simulink model "a_20210531_test_GPS"  (R2020b)
settings: Solver=FixedStepDiscrete  StartTime=0.0  StopTime=inf  FixedStep=0.01  RelTol=1e-3  EnableMultiTasking=on
libraries: arduinolib x2
settings Model: SimulationMode=external  SILPILModeSetting=veronly  ExtModeTrigDuration=2  Creator=alexv  LastModifiedBy=lapis-dspace
settings OptimizationCC: EnhancedBackFolding=on  PassReuseOutputArgsAs=Individual arguments  ZeroExternalMemoryAtStartup=off  ZeroInternalMemoryAtStartup=off  MaxStackSize=64  OptimizeBlockOrder=speed  DifferentSizesBufferReuse=on  OptimizationCustomize=off  EfficientTunableParamExpr=on
settings DebuggingCC: ParameterTunabilityLossMsg=error
settings HardwareCC: ProdBitPerPointer=32  ProdBitPerSizeT=32  ProdBitPerPtrDiffT=32  ProdLargestAtomicInteger=Long  ProdLargestAtomicFloat=Double  ProdWordSize=32  ProdHWDeviceType=ARM Compatible->ARM Cortex
settings SFSimCC: MATLABDynamicMemAlloc=off
settings RTWCC: Description=Embedded Coder  SystemTargetFile=ert.tlc  HardwareBoard=Arduino Due  TemplateMakefile=ert_default_tmf  Toolchain=Arduino ARM  BuildConfiguration=Faster Runs
settings CodeAppCC: ForceParamTrailComments=on  IgnoreCustomStorageClasses=off  OperatorAnnotations=on  SimulinkDataObjDesc=on  SFDataObjDesc=on  InsertBlockDesc=on
settings ERTTargetCC: SupportContinuousTime=on  SupportVariableSizeSignals=on  ExtModeTransport=3  ExtModeStaticAllocSize=24576  ExtModeMexFile=ext_xcp  ExtModeIntrfLevel=Level2 - Open

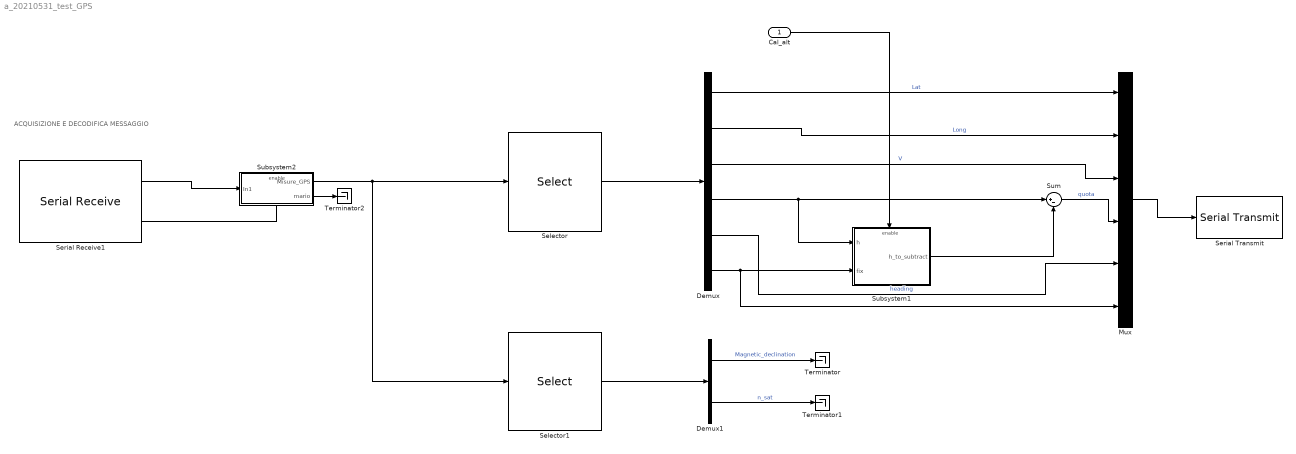
== system a_20210531_test_GPS ==
  note: ACQUISIZIONE E DECODIFICA MESSAGGIO
  Cal_alt : Inport
  Demux : Demux  Outputs=6
  Demux1 : Demux  Outputs=2
  Mux : Mux  Inputs=6
  Selector : Selector  InputPortWidth=9  IndexOptions=Index vector (dialog)  Indices=[1 2 3 8 5 6]  OutputSizes=1
  Selector1 : Selector  InputPortWidth=9  IndexOptions=Index vector (dialog)  Indices=[4 7]  OutputSizes=1
  Serial Receive1 : arduinolib/Serial Receive  isARMArch=on  portNumber=1  DataType=uint8  Datalength=32  SampleTime=0.01  showOutStatus=on  blockPlatform=arduino
      settings: SourceProductBaseCode=ARDUINO
  Serial Transmit : arduinolib/Serial Transmit  portNumber=0  sendmode=println  sendformat=Decimal  floatprecision=2  blockPlatform=arduino
  Subsystem1 : Subsystem
  Subsystem2 : Subsystem
  Sum : Sum  Inputs=|+-
  Terminator : Terminator
  Terminator1 : Terminator
  Terminator2 : Terminator
  wires:
  Demux1/2 -> Terminator1/1  "n_sat"
  Demux1/1 -> Terminator/1  "Magnetic_declination"
  Subsystem2/2(mario) -> Terminator2/1
  Selector/1 -> Demux/1
  Mux/1 -> Serial Transmit/1
  Demux/2 -> Mux/2  "Long"
  Sum/1 -> Mux/4  "quota"
  Serial Receive1/1 -> Subsystem2/1(In1)
  Cal_alt/1 -> Subsystem1/Enable
  Demux/3 -> Mux/3  "V"
  Demux/5 -> Mux/5  "heading"
  Subsystem1/1(h_to_subtract) -> Sum/2
  Selector1/1 -> Demux1/1
  Demux/1 -> Mux/1  "Lat"
  Demux/4 -> Sum/1, Subsystem1/1(h)
  Serial Receive1/2 -> Subsystem2/Enable
  Subsystem2/1(Misure_GPS) -> Selector/1, Selector1/1
  Demux/6 -> Mux/6, Subsystem1/2(fix)

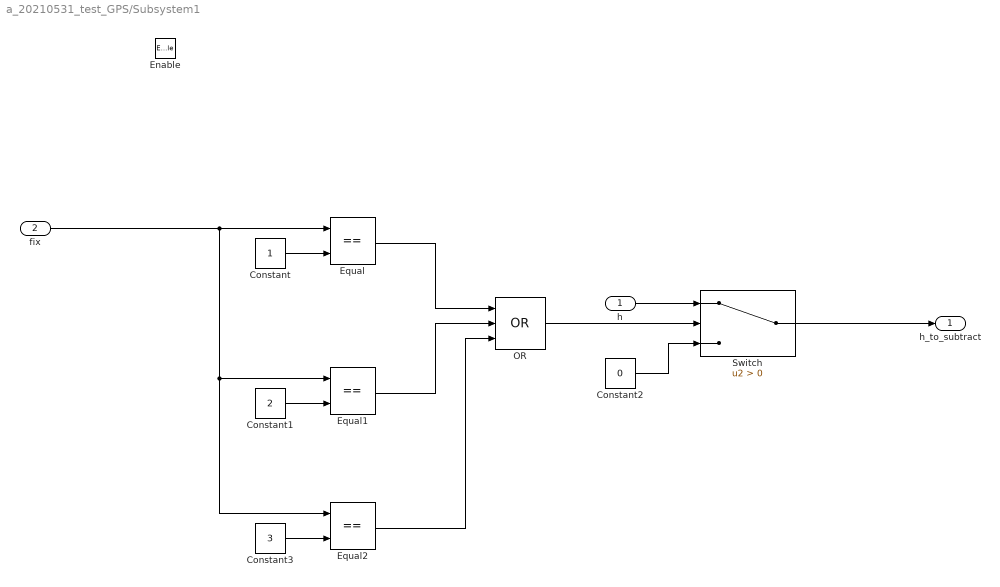
== system a_20210531_test_GPS/Subsystem1 ==
  h : Inport
  fix : Inport  Port=2
  Enable : EnablePort
  Constant : Constant
  Constant1 : Constant  Value=2
  Constant2 : Constant  Value=0
  Constant3 : Constant  Value=3
  Equal : RelationalOperator  Operator===  OutDataTypeStr=boolean  RndMeth=Simplest
  Equal1 : RelationalOperator  Operator===  OutDataTypeStr=boolean  RndMeth=Simplest
  Equal2 : RelationalOperator  Operator===  OutDataTypeStr=boolean  RndMeth=Simplest
  OR : Logic  Operator=OR  Inputs=3  IconShape=distinctive  AllPortsSameDT=off  OutDataTypeStr=boolean
  Switch : Switch  Criteria=u2 > Threshold
  h_to_subtract : Outport  VectorParamsAs1DForOutWhenUnconnected=off
  wires:
  Constant/1 -> Equal/2
  Equal/1 -> OR/1
  Constant1/1 -> Equal1/2
  Equal1/1 -> OR/2
  h/1 -> Switch/1
  OR/1 -> Switch/2
  Constant2/1 -> Switch/3
  Switch/1 -> h_to_subtract/1
  Equal2/1 -> OR/3
  Constant3/1 -> Equal2/2
  fix/1 -> Equal2/1, Equal1/1, Equal/1

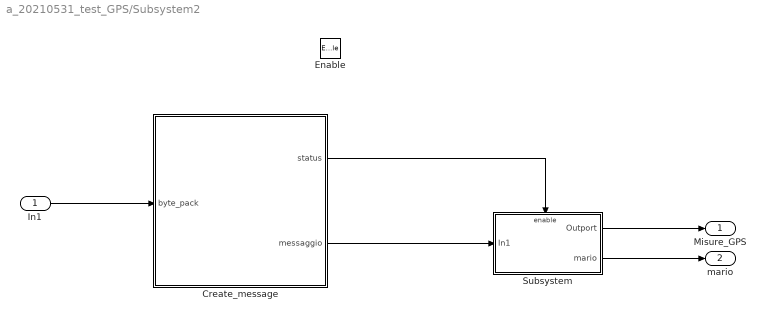
== system a_20210531_test_GPS/Subsystem2 ==
  In1 : Inport
  Enable : EnablePort
  Create_message : MATLAB Function  TreatAsAtomicUnit=on
  Subsystem : Subsystem
  Misure_GPS : Outport  VectorParamsAs1DForOutWhenUnconnected=off
  mario : Outport  Port=2  VectorParamsAs1DForOutWhenUnconnected=off
  wires:
  In1/1 -> Create_message/1(byte_pack)
  Create_message/1(status) -> Subsystem/Enable
  Subsystem/2(mario) -> mario/1
  Create_message/2(messaggio) -> Subsystem/1(In1)
  Subsystem/1(Outport) -> Misure_GPS/1

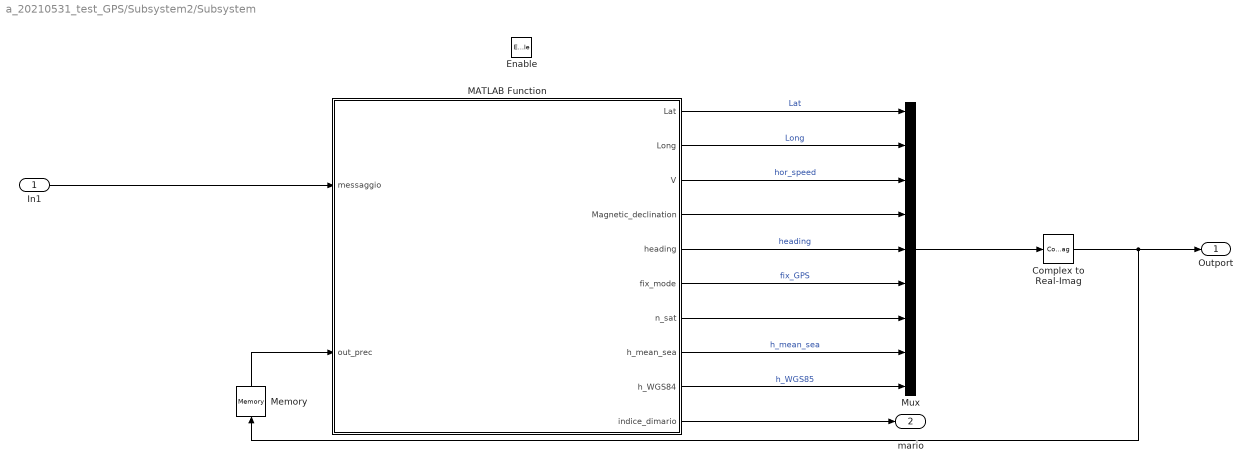
== system a_20210531_test_GPS/Subsystem2/Subsystem ==
  In1 : Inport
  Enable : EnablePort
  Complex to Real-Imag : ComplexToRealImag  Output=Real
  MATLAB Function : MATLAB Function  TreatAsAtomicUnit=on
  Memory : Memory  InheritSampleTime=on
  Mux : Mux  Inputs=9
  Outport : Outport  VectorParamsAs1DForOutWhenUnconnected=off
  mario : Outport  Port=2  VectorParamsAs1DForOutWhenUnconnected=off
  wires:
  MATLAB Function/2(Long) -> Mux/2  "Long"
  Memory/1 -> MATLAB Function/2(out_prec)
  MATLAB Function/8(h_mean_sea) -> Mux/8  "h_mean_sea"
  MATLAB Function/3(V) -> Mux/3  "hor_speed"
  MATLAB Function/1(Lat) -> Mux/1  "Lat"
  Mux/1 -> Complex to Real-Imag/1
  MATLAB Function/9(h_WGS84) -> Mux/9  "h_WGS85"
  MATLAB Function/5(heading) -> Mux/5  "heading"
  MATLAB Function/6(fix_mode) -> Mux/6  "fix_GPS"
  MATLAB Function/4(Magnetic_declination) -> Mux/4
  MATLAB Function/7(n_sat) -> Mux/7
  In1/1 -> MATLAB Function/1(messaggio)
  MATLAB Function/10(indice_dimario) -> mario/1
  Complex to Real-Imag/1 -> Memory/1, Outport/1

== matlab function a_20210531_test_GPS/Subsystem2/Create_message ==
  data: status output; byte_pack input; messaggio output
function [status,messaggio]  = LETTURA_NMEA(byte_pack)

persistent message counter start_found end_found

status = false;       %ho aggiunto questo
messaggio = uint8(zeros(1,80)) ;
pos_end = uint8(0) ;
M = uint8(length(byte_pack)) ;


if isempty(end_found) 
    end_found = false ;
end 
if isempty(start_found) 
     start_found = false ;
end 
if isempty (counter) 
    counter = uint8(0) ;
end 
if isempty(message)
     message = uint8(zeros(1,80)) ;
end



if start_found == 0 
    for i = uint8(1) : M  
        if byte_pack(i) == '$' 
            message(1:M - (i-1)) = byte_pack(i:end) ;
            counter = M - (i-1) ; 
            start_found = true ;
            break
        end
    end
    
    
elseif start_found == 1
    for i = uint8(1) : M  
        if byte_pack(i) == 13 
            end_found = true ;
            pos_end = i ;
            break
        end
    end
    
    if end_found == 1
        message(counter + 1 : counter + pos_end) = byte_pack(1:pos_end) ;
        status = true;       %ho aggiunto questo
        messaggio = message ;
        end_found = false ;
        counter = M - pos_end ;
        if pos_end == M 
            start_found = false ; 
            message = uint8(zeros(1,80)) ;
        else  
            start_found = true ;
            message(1:(M - pos_end)) = byte_pack(pos_end + 1 : end) ;
            message(M - pos_end +1 : 80) = uint8(zeros(1,80 - (M - pos_end) )) ;
        end
         

    else 
    message(counter + 1 : M + counter ) = byte_pack ;
    counter = M + counter  ;
   
    end
    
    
 
        
    
    
end

== matlab function a_20210531_test_GPS/Subsystem2/Subsystem/MATLAB Function ==
  data: messaggio input; Lat output; Long output; V output; Magnetic_declination output; heading output; fix_mode output; n_sat output; h_mean_sea output; h_WGS84 output; out_prec input; indice_dimario output
function [Lat,Long,V,Magnetic_declination,heading,fix_mode,n_sat,h_mean_sea,h_WGS84,indice_dimario] = parser_NMEA(messaggio,out_prec)


messaggio = char(messaggio) ;

comma_gga = uint8(zeros(1,14));
comma_rmc = uint8(zeros(1,12));
star = uint8(0);
dollar = uint8(0);
find_dollar = uint8(0);
find_comma = uint8(0);
message_type = uint8(zeros(1,5));
indice_dimario = uint8(0);





for i=1:length(messaggio)
    if messaggio(i) == '$'
        find_dollar = find_dollar + uint8(1);
    end
    if messaggio(i) == ','
        find_comma = find_comma + uint8(1);
    end
end

if (find_dollar == 1 && (find_comma == 12 || find_comma == 14))              % controllo se il numero di $ e , sono corretti all'interno di messaggio
    % altrimenti il messaggio è corrotto ed in output mando i messaggi
    % precedenti
    dollar= find(messaggio == '$',1);
    
    mess_type = messaggio(dollar(1) + 1 : dollar(1) + 5);                        % è il nome del messaggio arrivato
    
    % decodifica mesaggio RMC
    
    if mess_type == 'GPRMC'                                                          %esempio per i bimbi stupidi come noi: $GPRMC,081836,A,3751.65,S,14507.36,E,000.0,360.0,130998,011.3,E*62
        comma_rmc = find(messaggio == ',');                                          % restituisce le posizioni delle virgole all'interno del messaggio
        star = find(messaggio == '*');                                               % restituisce la posizione dell'asterisco all'interno del messaggio
        dollar = find(messaggio == '$');                                             % restituisce la posizione del dollaro all'interno del messaggio
        
        Lat_1 = str2double(messaggio(comma_rmc(3) + 1 : comma_rmc(3) + 2));
        Lat_2 = str2double(messaggio(comma_rmc(3) + 3 : comma_rmc(4) - 1))/60;
        Lat = Lat_1 + Lat_2;
        if messaggio(comma_rmc(4) + 1) == 'S'
            Lat = -Lat;
        end
        
        
        Long_1 = str2double(messaggio(comma_rmc(5) + 1 : comma_rmc(5) + 3));
        Long_2 = str2double(messaggio(comma_rmc(5) + 4 : comma_rmc(6) - 1))/60;
        Long = Long_1 + Long_2;
        if messaggio(comma_rmc(6) + 1) == 'W'
            Long = -Long;
        end
        
        V = str2double(messaggio(comma_rmc(7) + 1 : comma_rmc(8) - 1));
        
        heading = str2double(messaggio(comma_rmc(8) + 1 : comma_rmc(9) - 1));
        
        Magnetic_declination = str2double(messaggio(comma_rmc(10) + 1 : comma_rmc(11) - 1));
        if messaggio(comma_rmc(11) + 1) == 'W'
            Magnetic_declination = -Magnetic_declination;
        end
        
        % questi dati non sono presenti nel messaggio rmc, quindi prendo quelli
        % precedenti
        
        fix_mode = complex(out_prec(6),0);
        
        n_sat = complex(out_prec(7),0) ;
        
        h_mean_sea = complex(out_prec(8),0) ;
        
        h_WGS84 = complex(out_prec(9),0) ;
        
        
        %%%%%%%%%%%%%%%%%%%%%%%%%%%%%%%%%%%%%%%%%%%%%%%%%%%%%%%%%
        
        % calcolo checksum
        
        ck_ric = char(zeros(1,2)) ;
        ck_ric(1) = messaggio(star(1) + uint8(1))  ;
        ck_ric(2) = messaggio(star(1) + uint8(2)) ;
        
        NMEA_rmc_string = uint8(messaggio(dollar(1)+1:star(1)-1)) ;
        
        checksum = uint8(0) ;
        for i = 1:length(NMEA_rmc_string)
            checksum = bitxor(checksum,NMEA_rmc_string(i),'uint8') ;
        end
        
        if checksum ~= hex2dec(ck_ric)
            Lat = out_prec(1) ;
            Long = out_prec(2) ;
            V = out_prec(3) ;
            Magnetic_declination = out_prec(4);
            heading = out_prec(5) ;
            fix_mode = complex(out_prec(6),0);
            n_sat = complex(out_prec(7),0) ;
            h_mean_sea = complex(out_prec(8),0) ;
            h_WGS84 = complex(out_prec(9),0) ;
            indice_dimario = uint8(10);
        end
        
        %%%%%%%%%%%%%%%%%%%%%%%%%%%%%%%%%%%%%%%%%%%%%%%%%%%%%%%%%%%
        
        % decodifica mesaggio GGA
        
    elseif mess_type == 'GPGGA'
        comma_gga = find(messaggio == ',');
        star = find(messaggio == '*');
        dollar = find(messaggio == '$');
        
        
        Lat_1 = str2double(messaggio(comma_gga(2) + 1 : comma_gga(2) + 2));
        Lat_2 = str2double(messaggio(comma_gga(2) + 3 : comma_gga(3) - 1))/60;
        Lat = Lat_1 + Lat_2;
        if messaggio(comma_gga(3) + 1) == 'S'
            Lat = -Lat;
        end
        
        
        Long_1 = str2double(messaggio(comma_gga(4) + 1 : comma_gga(4) + 3));
        Long_2 = str2double(messaggio(comma_gga(4) + 4 : comma_gga(5) - 1))/60;
        Long = Long_1 + Long_2;
        if messaggio(comma_gga(5) + 1) == 'W'
            Long = -Long;
        end
        
        
        fix_mode = str2double(messaggio(comma_gga(6) + 1));
        
        n_sat = str2double(messaggio(comma_gga(7) + 1 : comma_gga(8) - 1));
        
        h_mean_sea = str2double(messaggio(comma_gga(9) + 1 : comma_gga(10) - 1));
        
        h_WGS84 = str2double(messaggio(comma_gga(11) + 1 : comma_gga(12) - 1));
        
        % questi dati non sono presenti nel messaggio rmc, quindi prendo quelli
        % precedenti
        
        V = out_prec(3) ;
        
        Magnetic_declination = out_prec(4);
        
        heading = out_prec(5) ;
        
        %%%%%%%%%%%%%%%%%%%%%%%%%%%%%%%%%%%%%%%%%%%%%%%%%%%%%%%%%%%%%%%%%%%
        
        % calcolo del checksum
        ck_ric = char(zeros(1,2)) ;
        ck_ric(1) = messaggio(star(1) + uint8(1))  ;
        ck_ric(2) = messaggio(star(1) + uint8(2)) ;
        
        NMEA_gga_string = uint8(messaggio(dollar(1)+1:star(1)-1)) ;
        
        checksum = uint8(0) ;
        for i = 1:length(NMEA_gga_string)
            checksum = bitxor(checksum,NMEA_gga_string(i),'uint8') ;
        end
        
        
        
        if checksum ~= hex2dec(ck_ric)
            Lat = out_prec(1) ;
            Long = out_prec(2) ;
            V = out_prec(3) ;
            Magnetic_declination = out_prec(4);
            heading = out_prec(5) ;
            fix_mode = complex(out_prec(6),0);
            
            n_sat = complex(out_prec(7),0) ;
            
            h_mean_sea = complex(out_prec(8),0) ;
            
            h_WGS84 = complex(out_prec(9),0) ;
            indice_dimario = uint8(20);
            
            
        end
        
        %%%%%%%%%%%%%%%%%%%%%%%%%%%%%%%%%%%%%%%%%%%%%%%%%%%%%%%%%%%%%%%%%%%%
        
    else
        
        Lat = out_prec(1) ;
        Long = out_prec(2) ;
        V = out_prec(3) ;
        Magnetic_declination = out_prec(4);
        heading = out_prec(5) ;
        fix_mode = complex(out_prec(6),0);
        
        n_sat = complex(out_prec(7),0) ;
        
        h_mean_sea = complex(out_prec(8),0) ;
        
        h_WGS84 = complex(out_prec(9),0) ;
        
        
        
    end
    
    
else
    
    Lat = out_prec(1) ;
    Long = out_prec(2) ;
    V = out_prec(3) ;
    Magnetic_declination = out_prec(4);
    heading = out_prec(5) ;
    fix_mode = complex(out_prec(6),0);
    n_sat = complex(out_prec(7),0) ;
    h_mean_sea = complex(out_prec(8),0) ;
    h_WGS84 = complex(out_prec(9),0) ;
end

end
